simulink model "AirFrame"  (R2025b)
settings: Solver=FixedStepAuto  StartTime=0.0  StopTime=10.0  RelTol=1e-3
settings Model: Creator=bohdanusatov  LastModifiedBy=bohdanusatov

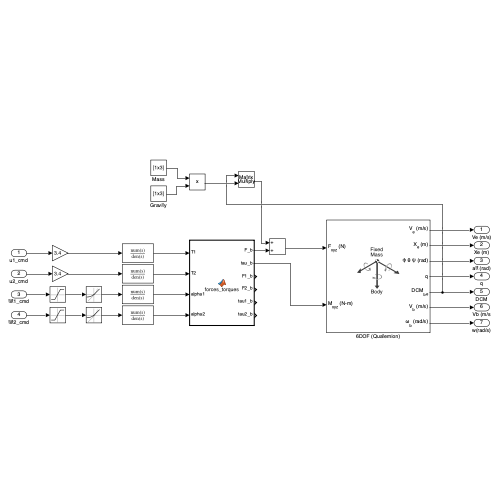
[thumbnail: Simulink's stored preview of the top-level diagram]
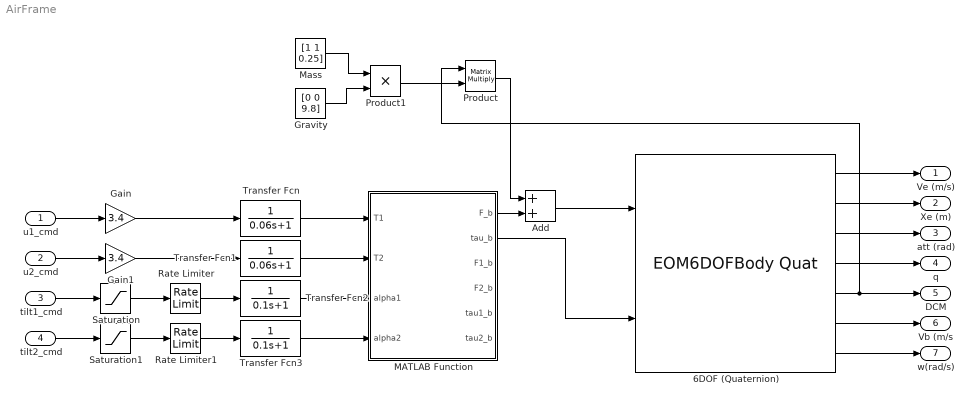
== system AirFrame ==
  u1_cmd : Inport
  u2_cmd : Inport  Port=2
  tilt1_cmd : Inport  Port=3
  tilt2_cmd : Inport  Port=4
  6DOF (Quaternion) : EOM6DOFBodyQuat  eul_0=[0.1 0 0]  mass_0=0.25
  Add : Sum
  Gain : Gain  Gain=3.4
  Gain1 : Gain  Gain=3.4
  Gravity : Constant  Value=[0 0 9.8]
  MATLAB Function : MATLAB Function  TreatAsAtomicUnit=on
  Mass : Constant  Value=[1 1 0.25]
  Product : Product  Multiplication=Matrix(*)
  Product1 : Product
  Rate Limiter : RateLimiter  RisingSlewLimit=8  FallingSlewLimit=-8  SampleTimeMode=inherited
  Rate Limiter1 : RateLimiter  RisingSlewLimit=8  FallingSlewLimit=-8  SampleTimeMode=inherited
  Saturation : Saturate  UpperLimit=0.35  LowerLimit=-0.35
  Saturation1 : Saturate  UpperLimit=0.35  LowerLimit=-0.35
  Transfer Fcn : TransferFcn  Denominator=[0.06 1]
  Transfer Fcn1 : TransferFcn  Denominator=[0.06 1]
  Transfer Fcn2 : TransferFcn  Denominator=[0.1 1]
  Transfer Fcn3 : TransferFcn  Denominator=[0.1 1]
  Ve (m/s) : Outport
  Xe (m) : Outport  Port=2
  att (rad) : Outport  Port=3
  q : Outport  Port=4
  DCM : Outport  Port=5
  Vb (m/s : Outport  Port=6
  w(rad/s) : Outport  Port=7
  wires:
  Product/1 -> Add/1
  Saturation/1 -> Rate Limiter/1
  Rate Limiter/1 -> Transfer Fcn2/1
  Transfer Fcn1/1 -> MATLAB Function/2(T2)
  MATLAB Function/1(F_b) -> Add/2
  Saturation1/1 -> Rate Limiter1/1
  Product1/1 -> Product/2
  6DOF (Quaternion)/5 -> DCM/1, Product/1
  Mass/1 -> Product1/1
  Transfer Fcn3/1 -> MATLAB Function/4(alpha2)
  Gain1/1 -> Transfer Fcn1/1
  Gravity/1 -> Product1/2
  Add/1 -> 6DOF (Quaternion)/1
  Gain/1 -> Transfer Fcn/1
  Transfer Fcn/1 -> MATLAB Function/1(T1)
  MATLAB Function/2(tau_b) -> 6DOF (Quaternion)/2
  Rate Limiter1/1 -> Transfer Fcn3/1
  Transfer Fcn2/1 -> MATLAB Function/3(alpha1)
  u1_cmd/1 -> Gain/1
  u2_cmd/1 -> Gain1/1
  tilt1_cmd/1 -> Saturation/1
  tilt2_cmd/1 -> Saturation1/1
  6DOF (Quaternion)/1 -> Ve (m/s)/1
  6DOF (Quaternion)/2 -> Xe (m)/1
  6DOF (Quaternion)/3 -> att (rad)/1
  6DOF (Quaternion)/4 -> q/1
  6DOF (Quaternion)/6 -> Vb (m/s/1
  6DOF (Quaternion)/7 -> w(rad/s)/1

== matlab function AirFrame/MATLAB Function ==
  data: F_b output; T1 input; T2 input; alpha1 input; alpha2 input; tau_b output; F1_b output; F2_b output; tau1_b output; tau2_b output
function [F_b, tau_b, F1_b, F2_b, tau1_b, tau2_b] = forces_torques(T1, T2, alpha1, alpha2)
% Minimal bicopter force/torque model (no Simscape)
%
% Assumptions:
% - Body axes: x forward, y right, z down (common autopilot body frame)
% - Rotors at r1=[0; +L; 0], r2=[0; -L; 0]
% - Tilt rotates thrust into x–z plane => rotation about +y axis
% - At alpha=0, thrust points along -z_b ("up" in z-down convention)
% - Positive alpha rotates thrust toward +x_b

% ---- parameters (edit) ----
L = 0.5;                  % [m] COM to rotor along +/-y
includeYawReaction = true;

% Very rough yaw reaction model (optional)
kQ_over_kT = 0.02;         % [-] only if includeYawReaction=true
spin1 = +1;                % rotor 1 spin direction (+1 or -1)
spin2 = -1;                % rotor 2 spin direction (+1 or -1)

% ---- rotor positions in body frame ----
r1 = [0; +L; 0];
r2 = [0; -L; 0];

% ---- thrust direction unit vectors in body frame ----
% Tilt about +y:
% alpha=0 -> [0; 0; -1]
% +alpha -> thrust gains +x component
t1_hat = [ sin(alpha1);
           0;
          -cos(alpha1) ];

t2_hat = [ sin(alpha2);
           0;
          -cos(alpha2) ];

% ---- rotor forces ----
F1_b = T1 * t1_hat;
F2_b = T2 * t2_hat;

F_b = F1_b + F2_b;

% ---- torques from moment arms ----
tau1_b = cross(r1, F1_b);
tau2_b = cross(r2, F2_b);

tau_b = tau1_b + tau2_b;

% ---- optional yaw reaction torque (very rough proxy) ----
if includeYawReaction
    tau_react_z = spin1 * kQ_over_kT * T1 + spin2 * kQ_over_kT * T2;
    tau_b = tau_b + [0; 0; tau_react_z];
end
end
